simulink model "MSE483_NonlinearSimulink"  (R2020b)
settings: Solver=ode113  StartTime=0.0  StopTime=10  RelTol=1e-3
InitFcn:
  | g = 9.81; %gravity
  | m = 0.03; % wheel weight
  | R = 0.04; % wheel radius
  | Jw = (m*R^2)/2; % wheel inertia moment
  | M = 0.6; % body weight
  | W = 0.14; % body width
  | D = 0.04; % body depth
  | H = 0.144; % body height
  | L = H/2; % distance to the CoM from wheel axel
  | J_psi = (M*L^2)/3; % body pitch inertia moment
  | J_phi = (M*(W^2 + D^2))/12; % body yaw inertia moment
  | Jm = 1E-5; % DC motor inertia moment
  | Rm = 6.69; % DC motor resistance
  | Kb = 0.468; % DC motor back EMF constant
  | Kt = 0.317; % DC motor torque constant
  | n = 1; % gear ratio
  | fm = 0.0022; % friction coefficient between body and motor
  | fw = 0; % friction coefficient between wheel and floor
  | f_w = 0;
  | 
  | a = (n*Kt)/Rm;
  | b = ((n*Kt*Kb)/Rm) + fm;
  | 
  | 
  | A=[0,  0,           1,          0;
  |     0,  0,           0,          1;
  |     0, -409.7184,  -104.6299,   104.6299;
  |     0,  268.6273,    54.5833,   -54.5833]
  | B = [0;0;101.6952;-53.0523]
  | C=[1,0,0,0;]
  | D=[0]
  | x0=[0;90*pi/180;0;0]
  | K=[-318.517516293979	-839.316963783976	-66.2263834004483	-127.491021126397]
  | KI = 890.808276084874
  | Ob= [ 400.0000   ,      0   , 1.0000  ,       0;
  |          0 , 400.0000   ,      0  ,  1.0000;
  |          0, -409.718, 295.3701 , 104.6299;
  |          0,  268.6273 ,  54.5833 , 345.4167]
settings Model: Creator=Sepehrrf  LastModifiedBy=mkupp
settings SolverCC: AlgebraicLoopSolver=LineSearch

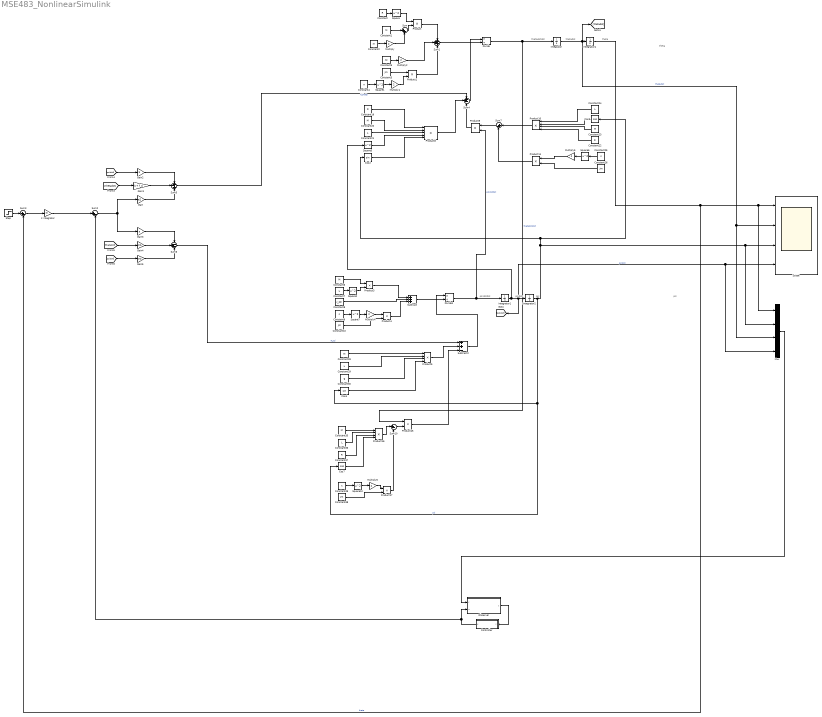
== system MSE483_NonlinearSimulink ==
  note: psi
  note: thetadotdot
  note: psidot
  note: thetadot
  note: psidotdot
  note: psi
  note: theta
  note: theta
  Constant{,19,22,37} (4 alike) : Constant  Value=R
  Constant{1,6,20,23,28,35} (6 alike) : Constant  Value=M
  Constant{3,10,26,38} (4 alike) : Constant  Value=Jm
  Constant2 : Constant  Value=m
  Constant{7,21,24,29,36} (5 alike) : Constant  Value=L
  Constant{4,9,25,39} (4 alike) : Constant  Value=n
  Constant30 : Constant  Value=g
  Constant5 : Constant  Value=Jw
  Constant8 : Constant  Value=J_psi
  Controller : Subsystem
  Cos2 : Trigonometry
  Cos3 : Trigonometry  Operator=cos
  Cos4 : Trigonometry
  Cos7 : Trigonometry  Operator=cos
  Divide : Product  Inputs=*/
  Divide1 : Product  Inputs=*/
  Gain : Gain  Gain=a/2
  Gain1 : Gain  Gain=b + f_w
  Gain2 : Gain  Gain=b
  Gain3 : Gain  Gain=a
  Gain4 : Gain  Gain=2*b
  Gain5 : Gain  Gain=2*b
  Integrator : Integrator
  Integrator1 : Integrator
  Integrator2 : Integrator  InitialCondition=0.1
  Integrator4 : Integrator
  K integrator : Gain  InitFcn=|  Gain=KI
      | A=[0,  0,           1,          0;
      |     0,  0,           0,          1;
      |     0, -409.7184,  -104.6299,   104.6299;
      |     0,  268.6273,    54.5833,   -54.5833]
      | B = [0;0;101.6952;-53.0523]
      | C=[1 0 0 0]
      | D=[0]
      | x0=[0;90*pi/180;0;0]
      | K=[-62.8966122663488	-201.905572339641	-14.9133345772124	-27.6218237282572]
      | Ob= [ 400.0000   ,      0   , 1.0000  ,       0;
      |          0 , 400.0000   ,      0  ,  1.0000;
      |          0, -409.718, 295.3701 , 104.6299;
      |          0,  268.6273 ,  54.5833 , 345.4167]
  Multiply{,1..2,4..6} (6 alike) : Gain  Gain=2
  Mux : Mux
  Observer : Subsystem
  Product{,1,3..4,9,11,15,17} (8 alike) : Product
  Product10 : Product  Inputs=4
  Product16 : Product  Inputs=4
  Product5 : Product  Inputs=4
  Product8 : Product  Inputs=5
  Scope : Scope  NumInputPorts=4
  Square{,1..2,5..7,10} (7 alike) : Math  Operator=square  SignedPower=on  RndMeth=Zero  SaturateOnIntegerOverflow=on
  Step : Step  SampleTime=0
  Subtract : Sum  Inputs=+++
  Subtract2 : Sum  Inputs=++-
  Sum : Sum  Inputs=|++
  Sum1 : Sum  Inputs=+++
  Sum{2..3,7,10} (4 alike) : Sum  Inputs=|+-
  Sum4 : Sum  Inputs=++-
  Sum5 : Sum  Inputs=+-+
  Sum6 : Sum  Inputs=-+-
  wires:
  Constant/1 -> Square/1
  Square5/1 -> Product8/4
  Constant4/1 -> Square1/1
  Cos2/1 -> Product8/5
  Square1/1 -> Multiply1/1
  Constant2/1 -> Multiply/1
  Integrator4/1 -> Scope/1, Mux/1, Sum3/2  "theta"
  Constant21/1 -> Product8/3
  Product17/1 -> Sum10/2
  Multiply1/1 -> Product1/2
  Product16/1 -> Sum10/1
  Constant1/1 -> Sum/1
  Multiply/1 -> Sum/2
  Constant22/1 -> Product10/4
  Product4/1 -> Subtract/3
  Constant39/1 -> Square10/1
  Constant20/1 -> Product8/2
  Integrator1/1 -> Square5/1, [psidot], Mux/4, Scope/4, Integrator2/1  "psidot"
  Product/1 -> Sum1/1
  Constant3/1 -> Product1/1
  Constant5/1 -> Multiply2/1
  Sum1/1 -> Divide/2
  Product8/1 -> Sum4/2
  Constant10/1 -> Product4/2
  Divide/1 -> Integrator/1, Product15/1  "thetadotdot"
  Constant19/1 -> Product8/1
  Product3/1 -> Subtract/1
  Multiply2/1 -> Sum1/2
  Product1/1 -> Sum1/3
  Constant38/1 -> Product17/2
  Integrator2/1 -> Cos7/1, Cos4/1, Mux/2, Scope/3, Cos3/1, Cos2/1  "psi"
  Square6/1 -> Multiply5/1
  Product9/1 -> Sum4/3
  Constant25/1 -> Square6/1
  Divide1/1 -> Product9/2, Integrator1/1  "psidotdot"
  Square7/1 -> Multiply4/1
  Product10/1 -> Sum7/1
  Square10/1 -> Multiply6/1
  Constant35/1 -> Product16/1
  Sum/1 -> Product/2
  Cos3/1 -> Product10/2
  Constant7/1 -> Square2/1
  Constant23/1 -> Product10/3
  Constant6/1 -> Product3/1
  Product11/1 -> Sum7/2
  Constant8/1 -> Subtract/2
  Square2/1 -> Product3/2
  Multiply5/1 -> Product11/1
  Constant30/1 -> Product5/3
  Constant36/1 -> Product16/2
  Constant28/1 -> Product5/1
  Square/1 -> Product/1
  Constant37/1 -> Product16/3
  Integrator/1 -> [thetadot], Mux/3, Scope/2, Integrator4/1  "thetadot"
  Sum7/1 -> Product9/1
  Constant24/1 -> Product10/1
  Constant9/1 -> Square7/1
  Subtract/1 -> Divide1/2
  Multiply4/1 -> Product4/1
  Subtract2/1 -> Divide1/1
  Product5/1 -> Subtract2/2
  Multiply6/1 -> Product17/1
  Cos7/1 -> Product16/4
  Sum10/1 -> Product15/2
  Constant26/1 -> Product11/2
  Sum4/1 -> Divide/1
  Constant29/1 -> Product5/2
  Cos4/1 -> Product5/4
  Product15/1 -> Subtract2/3
  [thetadot] -> Gain1/1
  Sum6/1 -> Subtract2/1  "F_psi"
  Gain4/1 -> Sum6/2
  Sum5/1 -> Sum4/1  "F_theta"
  Gain3/1 -> Sum6/1
  [thetadot] -> Gain4/1
  [psidot] -> Gain2/1
  [psidot] -> Gain5/1
  Gain1/1 -> Sum5/2
  Gain5/1 -> Sum6/3
  Gain2/1 -> Sum5/1
  Gain/1 -> Sum5/3
  Mux/1 -> Observer/1(y)
  Observer/1(x) -> Controller/1(x)
  Controller/1(u) -> Sum2/2, Observer/2(u)
  K integrator/1 -> Sum2/1
  Sum2/1 -> Gain3/1, Gain/1
  Sum3/1 -> K integrator/1
  Step/1 -> Sum3/1

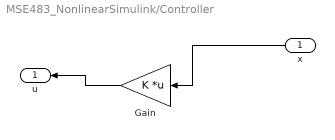
== system MSE483_NonlinearSimulink/Controller ==
  x : Inport
  Gain : Gain  Gain=K  Multiplication=Matrix(K*u)
  u : Outport
  wires:
  Gain/1 -> u/1
  x/1 -> Gain/1

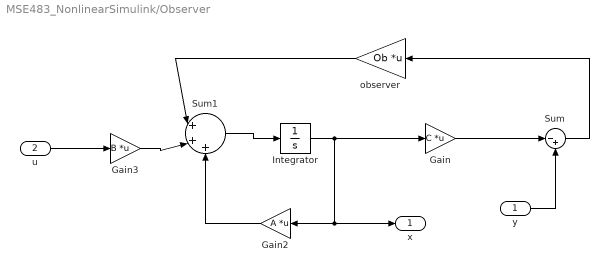
== system MSE483_NonlinearSimulink/Observer ==
  y : Inport
  u : Inport  Port=2
  Gain : Gain  Gain=C  Multiplication=Matrix(K*u)
  Gain2 : Gain  Gain=A  Multiplication=Matrix(K*u)
  Gain3 : Gain  Gain=B  Multiplication=Matrix(K*u)
  Integrator : Integrator  InitialCondition=x0
  Sum : Sum  Inputs=|-+
  Sum1 : Sum  Inputs=|+++
  observer : Gain  Gain=Ob  Multiplication=Matrix(K*u)
  x : Outport
  wires:
  u/1 -> Gain3/1
  Gain/1 -> Sum/1
  Sum1/1 -> Integrator/1
  Integrator/1 -> Gain2/1, x/1, Gain/1
  y/1 -> Sum/2
  Sum/1 -> observer/1
  observer/1 -> Sum1/1
  Gain3/1 -> Sum1/2
  Gain2/1 -> Sum1/3
